simulink model "PolePlaceHeliInteger"  (R2021a)
settings: Solver=VariableStepAuto  StartTime=0.0  StopTime=10.0  MaxStep=1e-3  RelTol=1e-3
values from neighbouring files (symbols this model uses):
  A = [0 0 1 0 ... (first row only)    [HeliControlGain.m]    (also in HeliControlHinf.m; HeliControlInteger.m; HeliControlLQG.m; HeliControlLQRgain.m)
  B = [0 0 ... (first row only)    [HeliControlGain.m]    (also in HeliControlHinf.m; HeliControlInteger.m; HeliControlLQG.m; HeliControlLQRgain.m)
  C = [1 0 0 0 ... (first row only)    [HeliControlGain.m]    (also in HeliControlHinf.m; HeliControlInteger.m; HeliControlLQG.m; HeliControlLQRgain.m)
  Kf = K(:,1:4)    [HeliControlInteger.m]    (also in HeliControlIntegerObsv.m; HeliControlLQG.m; HeliControlLQRinteger.m)
  Ki = K(:,5:end)    [HeliControlInteger.m]    (also in HeliControlIntegerObsv.m; HeliControlLQG.m; HeliControlLQRinteger.m)
settings Model: Creator=Ciro  LastModifiedBy=Ciro

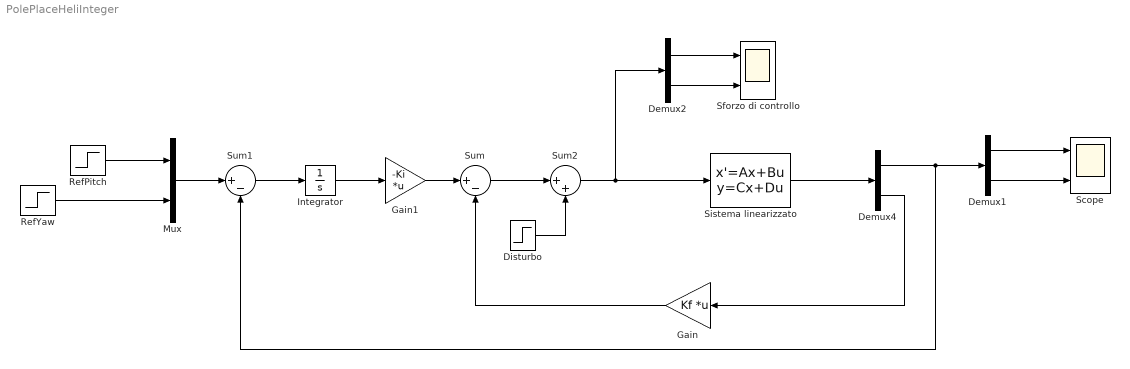
== system PolePlaceHeliInteger ==
  Demux1 : Demux  Outputs=2
  Demux2 : Demux  Outputs=2
  Demux4 : Demux  Outputs=[2 4]
  Disturbo : Step  Time=6  After=0  SampleTime=0
  Gain : Gain  Gain=Kf  Multiplication=Matrix(K*u)
  Gain1 : Gain  Gain=-Ki  Multiplication=Matrix(K*u)
  Integrator : Integrator
  Mux : Mux  Inputs=2
  RefPitch : Step  After=0.3  SampleTime=0
  RefYaw : Step  After=0.3  SampleTime=0
  Scope : Scope  NumInputPorts=2
  Sforzo di controllo : Scope  NumInputPorts=2
  Sistema linearizzato : StateSpace  A=A  B=B  C=[C; eye(4)]  D=zeros(6,2)  InitialCondition=[0;0;0;0]  ParameterTunability=Optimized
  Sum : Sum  Inputs=|+-
  Sum1 : Sum  Inputs=|+-
  Sum2 : Sum  Inputs=|++
  wires:
  Gain/1 -> Sum/2
  RefPitch/1 -> Mux/1
  RefYaw/1 -> Mux/2
  Gain1/1 -> Sum/1
  Demux2/1 -> Sforzo di controllo/1
  Demux2/2 -> Sforzo di controllo/2
  Sum/1 -> Sum2/1
  Sum2/1 -> Demux2/1, Sistema linearizzato/1
  Disturbo/1 -> Sum2/2
  Sistema linearizzato/1 -> Demux4/1
  Demux4/2 -> Gain/1
  Demux1/1 -> Scope/1
  Demux1/2 -> Scope/2
  Demux4/1 -> Sum1/2, Demux1/1
  Integrator/1 -> Gain1/1
  Mux/1 -> Sum1/1
  Sum1/1 -> Integrator/1
